simulink model "quadrupleTankNLMPC"  (R2023a)
settings: Solver=VariableStepAuto  StartTime=0.0  StopTime=300  RelTol=1e-3
values from neighbouring files (symbols this model uses):
  us = [37,38]'    [ControlOfQuadrupletankUsingPassivityBasedNonlinearMPC1.m]    (also in getPassivityInputQuadrupleTank.m; getPassivityOutputQuadrupleTank.m)
  x0 = [25;16;20;21]    [ControlOfQuadrupletankUsingPassivityBasedNonlinearMPC1.m]
  xs = [28.1459,17.8230,18.3991,25.1192]'    [ControlOfQuadrupletankUsingPassivityBasedNonlinearMPC1.m]    (also in getPassivityInputQuadrupleTank.m; getPassivityOutputQuadrupleTank.m)
libraries: mpclib x1
settings Model: Creator=The MathWorks, Inc.  LastModifiedBy=The MathWorks, Inc.
settings SolverCC: MaxZcPerStep=1
settings OptimizationCC: ReuseModelBlockBuffer=off
settings DebuggingCC: UnconnectedInputMsg=warning  UnconnectedOutputMsg=warning  UnconnectedLineMsg=warning
settings ModelReferenceCC: EnableRefExpFcnMdlSchedulingChecks=on
settings RTWCC: DLArmComputeVersion=19.05

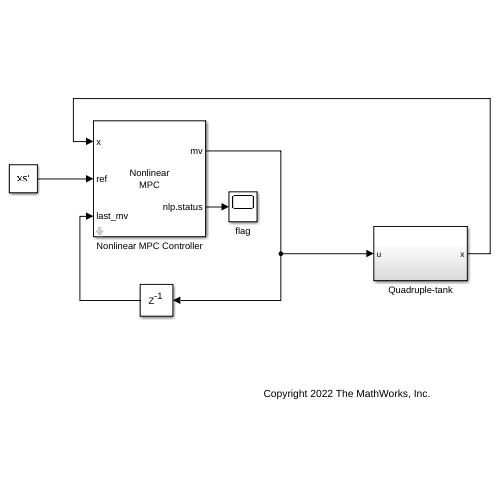
[thumbnail: Simulink's stored preview of the top-level diagram]
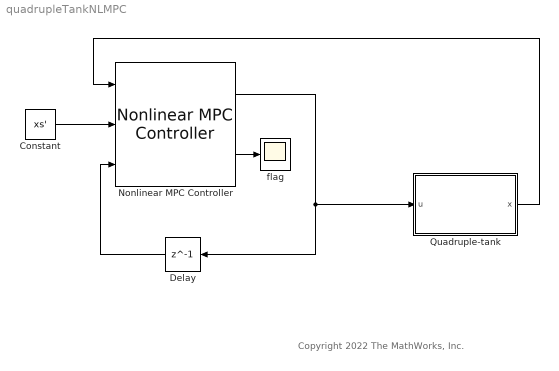
== system quadrupleTankNLMPC ==
  note: Copyright 2022 The MathWorks, Inc.
  Constant : Constant  Value=xs'  VectorParams1D=off
  Delay : Delay  DelayLength=1  InitialCondition=0
  Nonlinear MPC Controller : mpclib/Nonlinear MPC Controller  nlmpcobj=nlobj  UseObjectTs=on  UseMEX=off  md_enabled=off  mvtarget_enabled=off  param_enabled=off  cost_enabled=off  mvseq_enabled=off  stateseq_enabled=off  ovseq_enabled=off  slack_enabled=off  status_enabled=on  ov_min=off  ov_max=off  mv_min=off  mv_max=off  mvrate_min=off  mvrate_max=off  state_min=off  state_max=off  ov_weight=off  mv_weight=off  mvrate_weight=off  ecr_weight=off  nlp_initialize=off
  Quadruple-tank : Subsystem
  flag : Scope
  wires:
  Constant/1 -> Nonlinear MPC Controller/2
  Nonlinear MPC Controller/1 -> Delay/1, Quadruple-tank/1(u)
  Delay/1 -> Nonlinear MPC Controller/3
  Quadruple-tank/1(x) -> Nonlinear MPC Controller/1
  Nonlinear MPC Controller/2 -> flag/1

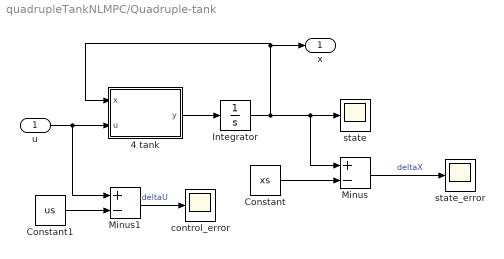
== system quadrupleTankNLMPC/Quadruple-tank ==
  u : Inport
  4 tank : MATLAB Function  TreatAsAtomicUnit=on
  Constant : Constant  Value=xs  VectorParams1D=off
  Constant1 : Constant  Value=us  VectorParams1D=off
  Integrator : Integrator  InitialCondition=x0
  Minus : Sum  Inputs=+-
  Minus1 : Sum  Inputs=+-
  control_error : Scope
  state : Scope
  state_error : Scope
  x : Outport
  wires:
  Integrator/1 -> Minus/1, state/1, 4 tank/1(x), x/1
  u/1 -> Minus1/1, 4 tank/2(u)
  4 tank/1(y) -> Integrator/1
  Constant/1 -> Minus/2
  Minus/1 -> state_error/1  "deltaX"
  Constant1/1 -> Minus1/2
  Minus1/1 -> control_error/1  "deltaU"

== matlab function quadrupleTankNLMPC/Quadruple-tank/4 tank ==
  data: x input; u input; y output
function y = fcn(x,u)

y = stateFcnQuadrupleTank(x,u);
